simulink model "simpleOrientationSim"  (R2015a)
settings: Solver=ode45  StartTime=0.0  StopTime=10.0  RelTol=1e-3
values from neighbouring files (symbols this model uses):
  K_lqr = lqr(A,B,Q,R)    [OrientationLQR.m]
settings Model: Creator=ra  LastModifiedBy=ra

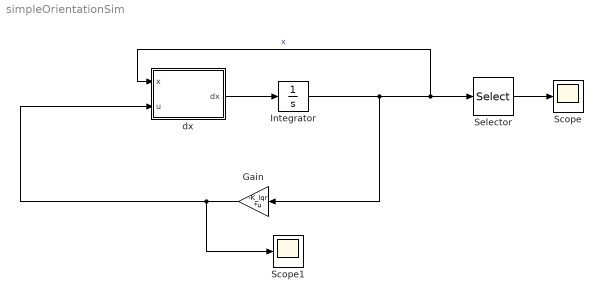
== system simpleOrientationSim ==
  Gain : Gain  Gain=-K_lqr  Multiplication=Matrix(K*u)
  Integrator : Integrator  InitialCondition=[0.175 0.175 0.175 1 1 0.1]
  Scope : Scope
  Scope1 : Scope
  Selector : Selector  InputPortWidth=6  Indices=[1:3]
  dx : MATLAB Function  TreatAsAtomicUnit=on
  wires:
  dx/1(dx) -> Integrator/1
  Integrator/1 -> Gain/1, Selector/1, dx/1(x)  "x"
  Gain/1 -> Scope1/1, dx/2(u)
  Selector/1 -> Scope/1

== matlab function simpleOrientationSim/dx ==
  data: x input; u input; dx output
function dx = fcn(x,u)
yaw=x(1);
pitch=x(2);
roll=x(3);
p=x(4);
q=x(5);
r=x(6);

taur = u(1);
taup = u(2);
tauy = u(3);

Jxs = 0.0058;
Jys = 0.0058;
Jzs = 0.0104;

dx = zeros(6,1);

 dx(1) = (r*cos(roll))/cos(pitch) + (q*sin(roll))/cos(pitch);
 dx(2) = q*cos(roll) - r*sin(roll);
 dx(3) = p + (r*cos(roll)*sin(pitch))/cos(pitch) + (q*sin(pitch)*sin(roll))/cos(pitch);
 

 dx(4) = (taur + Jys*q*r - Jzs*q*r)/Jxs;
 dx(5) = (taup - Jxs*p*r + Jzs*p*r)/Jys;
 dx(6) = (tauy + Jxs*p*q - Jys*p*q)/Jzs;
